simulink model "Marine_LocoMotive_UAV_est_git"  (R2018a)
settings: Solver=ode4  StartTime=0.0  StopTime=40  FixedStep=T  MaxStep=2*T  MinStep=T  RelTol=1e-4
values from neighbouring files (symbols this model uses):
  a_11 = 0.05*m_b    (= 0.625)    [Marine_LocoMotive_UAV_est_git_parameters.m]    (also in Marine_LocoMotive_UAV_medium_est_git_parameters.m = 1.6875; heave_dynamics_chart.m)
  a_33 = m_b    (= 12.5)    [Marine_LocoMotive_UAV_est_git_parameters.m]    (also in Marine_LocoMotive_UAV_medium_est_git_parameters.m = 33.75; heave_dynamics_chart.m)
  A_w = 1*3.3/2    (= 1.65)    [Marine_LocoMotive_UAV_est_git_parameters.m]    (also in Marine_LocoMotive_UAV_medium_est_git_parameters.m = 0.6)
  A_w2 = 1*1.2/2    (= 0.6)    [Marine_LocoMotive_UAV_est_git_parameters.m]    (also in Marine_LocoMotive_UAV_medium_est_git_parameters.m = 0.305)
  Ac = 0.0331    [Marine_LocoMotive_UAV_est_git_parameters.m]    (also in Marine_LocoMotive_UAV_medium_est_git_parameters.m = 0.422)
  alpha_bar = pi/4    (= 0.785398163397)    [Marine_LocoMotive_UAV_est_git_parameters.m]    (also in Marine_LocoMotive_UAV_medium_est_git_parameters.m; heave_dynamics_chart.m = pi/4*sign(V_bar(j)))
  Am = sysd.denominator{1}    [Marine_LocoMotive_UAV_est_git_parameters.m]    (also in Marine_LocoMotive_UAV_medium_est_git_parameters.m)
  Am1_LPF = sysd.denominator{1}    [Marine_LocoMotive_UAV_est_git_parameters.m]    (also in Marine_LocoMotive_UAV_medium_est_git_parameters.m)
  Am2_LPF = sysd.denominator{1}    [Marine_LocoMotive_UAV_est_git_parameters.m]    (also in Marine_LocoMotive_UAV_medium_est_git_parameters.m)
  Am_asw_LPF = sysd.denominator{1}    [Marine_LocoMotive_UAV_est_git_parameters.m]    (also in Marine_LocoMotive_UAV_medium_est_git_parameters.m)
  Am_coup_LPF = sysd.denominator{1}    [Marine_LocoMotive_UAV_est_git_parameters.m]    (also in Marine_LocoMotive_UAV_medium_est_git_parameters.m)
  Am_fast_coup_LPF = sysd.denominator{1}    [Marine_LocoMotive_UAV_est_git_parameters.m]    (also in Marine_LocoMotive_UAV_medium_est_git_parameters.m)
  Am_rdeL_LPF = sysd.denominator{1}    [Marine_LocoMotive_UAV_est_git_parameters.m]    (also in Marine_LocoMotive_UAV_medium_est_git_parameters.m)
  Am_reL_LPF = sysd.denominator{1}    [Marine_LocoMotive_UAV_est_git_parameters.m]    (also in Marine_LocoMotive_UAV_medium_est_git_parameters.m)
  Am_rref20_LPF = sysd.denominator{1}    [Marine_LocoMotive_UAV_est_git_parameters.m]    (also in Marine_LocoMotive_UAV_medium_est_git_parameters.m)
  Am_rref_LPF = sysd.denominator{1}    [Marine_LocoMotive_UAV_est_git_parameters.m]    (also in Marine_LocoMotive_UAV_medium_est_git_parameters.m)
  AmAlpha_LPF = sysd.denominator{1}    [Marine_LocoMotive_UAV_est_git_parameters.m]    (also in Marine_LocoMotive_UAV_medium_est_git_parameters.m)
  Amp_sf = 3    [Marine_LocoMotive_UAV_est_git_parameters.m]    (also in Marine_LocoMotive_UAV_medium_est_git_parameters.m)
  Amp_sf_rp = 0.05*m_u*g    (= 0.8829)    [Marine_LocoMotive_UAV_est_git_parameters.m]    (also in Marine_LocoMotive_UAV_medium_est_git_parameters.m = 9.56475)
  AmV_LPF = sysd.denominator{1}    [Marine_LocoMotive_UAV_est_git_parameters.m]    (also in Marine_LocoMotive_UAV_medium_est_git_parameters.m)
  AmZ_LPF = sysd.denominator{1}    [Marine_LocoMotive_UAV_est_git_parameters.m]    (also in Marine_LocoMotive_UAV_medium_est_git_parameters.m)
  b_11 = 0    [Marine_LocoMotive_UAV_est_git_parameters.m]    (also in Marine_LocoMotive_UAV_medium_est_git_parameters.m; heave_dynamics_chart.m)
  b_33 = 2*m_b*omega_h    (= 19.6349540849)    [Marine_LocoMotive_UAV_est_git_parameters.m]    (also in Marine_LocoMotive_UAV_medium_est_git_parameters.m = 84.8230016469; buoyancy_calc.m = 4.18879020479; heave_dynamics_chart.m = 2*m_b*omega_h)
  Bm = sysd.numerator{1}    [Marine_LocoMotive_UAV_est_git_parameters.m]    (also in Marine_LocoMotive_UAV_medium_est_git_parameters.m)
  Bm1_LPF = sysd.numerator{1}    [Marine_LocoMotive_UAV_est_git_parameters.m]    (also in Marine_LocoMotive_UAV_medium_est_git_parameters.m)
  Bm2_LPF = sysd.numerator{1}    [Marine_LocoMotive_UAV_est_git_parameters.m]    (also in Marine_LocoMotive_UAV_medium_est_git_parameters.m)
  Bm_asw_LPF = sysd.numerator{1}    [Marine_LocoMotive_UAV_est_git_parameters.m]    (also in Marine_LocoMotive_UAV_medium_est_git_parameters.m)
  Bm_coup_LPF = sysd.numerator{1}    [Marine_LocoMotive_UAV_est_git_parameters.m]    (also in Marine_LocoMotive_UAV_medium_est_git_parameters.m)
  Bm_fast_coup_LPF = sysd.numerator{1}    [Marine_LocoMotive_UAV_est_git_parameters.m]    (also in Marine_LocoMotive_UAV_medium_est_git_parameters.m)
  Bm_rdeL_LPF = sysd.numerator{1}    [Marine_LocoMotive_UAV_est_git_parameters.m]    (also in Marine_LocoMotive_UAV_medium_est_git_parameters.m)
  Bm_reL_LPF = sysd.numerator{1}    [Marine_LocoMotive_UAV_est_git_parameters.m]    (also in Marine_LocoMotive_UAV_medium_est_git_parameters.m)
  Bm_rref20_LPF = sysd.numerator{1}    [Marine_LocoMotive_UAV_est_git_parameters.m]    (also in Marine_LocoMotive_UAV_medium_est_git_parameters.m)
  Bm_rref_LPF = sysd.numerator{1}    [Marine_LocoMotive_UAV_est_git_parameters.m]    (also in Marine_LocoMotive_UAV_medium_est_git_parameters.m)
  BmAlpha_LPF = sysd.numerator{1}    [Marine_LocoMotive_UAV_est_git_parameters.m]    (also in Marine_LocoMotive_UAV_medium_est_git_parameters.m)
  BmV_LPF = sysd.numerator{1}    [Marine_LocoMotive_UAV_est_git_parameters.m]    (also in Marine_LocoMotive_UAV_medium_est_git_parameters.m)
  BmZ_LPF = sysd.numerator{1}    [Marine_LocoMotive_UAV_est_git_parameters.m]    (also in Marine_LocoMotive_UAV_medium_est_git_parameters.m)
  C_S = [5;9]*10^-3    [Marine_LocoMotive_UAV_est_git_parameters.m]    (also in Marine_LocoMotive_UAV_medium_est_git_parameters.m; heave_dynamics_chart.m = 0.075/(log10(Re)-2)^2)
  Cd_u = 0.2    [Marine_LocoMotive_UAV_est_git_parameters.m]    (also in Marine_LocoMotive_UAV_medium_est_git_parameters.m)
  D_x = b_11 + D_s(1)    [Marine_LocoMotive_UAV_est_git_parameters.m]    (also in Marine_LocoMotive_UAV_medium_est_git_parameters.m; heave_dynamics_chart.m = b_11 + D_s(i,j))
  D_z = b_33 + D_s(2)    [Marine_LocoMotive_UAV_est_git_parameters.m]    (also in Marine_LocoMotive_UAV_medium_est_git_parameters.m; heave_dynamics_chart.m)
  dc_M_p = 6.7    [Marine_LocoMotive_UAV_est_git_parameters.m]    (also in Marine_LocoMotive_UAV_medium_est_git_parameters.m)
  Delta_h = (A_im/A_b-0.5)*h_b    (= -0.0625)    [Marine_LocoMotive_UAV_est_git_parameters.m]    (also in Marine_LocoMotive_UAV_medium_est_git_parameters.m = -0.075; heave_dynamics_chart.m)
  eps_V = 0.1    [Marine_LocoMotive_UAV_est_git_parameters.m]    (also in Marine_LocoMotive_UAV_medium_est_git_parameters.m)
  epsilon_1 = 5    [Marine_LocoMotive_UAV_est_git_parameters.m]    (also in Marine_LocoMotive_UAV_medium_est_git_parameters.m)
  epsilon_e_u1 = 0.05    [Marine_LocoMotive_UAV_est_git_parameters.m]    (also in Marine_LocoMotive_UAV_medium_est_git_parameters.m)
  epsilon_w = 0    [Marine_LocoMotive_UAV_est_git_parameters.m]    (also in Marine_LocoMotive_UAV_medium_est_git_parameters.m)
  epsilon_w2 = pi    (= 3.14159265359)    [Marine_LocoMotive_UAV_est_git_parameters.m]    (also in Marine_LocoMotive_UAV_medium_est_git_parameters.m)
  g = 9.81    [Marine_LocoMotive_UAV_est_git_parameters.m]    (also in Marine_LocoMotive_UAV_medium_est_git_parameters.m; heave_dynamics_chart.m)
  gamma_d_p = (2*0.3/0.03*2*0.2*12/4)/10    (= 2.4)    [Marine_LocoMotive_UAV_est_git_parameters.m]    (also in Marine_LocoMotive_UAV_medium_est_git_parameters.m)
  H = 10    [Marine_LocoMotive_UAV_est_git_parameters.m]    (also in Marine_LocoMotive_UAV_medium_est_git_parameters.m)
  h_b = 0.25    [Marine_LocoMotive_UAV_est_git_parameters.m]    (also in Marine_LocoMotive_UAV_medium_est_git_parameters.m = 0.3; buoyancy_calc.m = 0.15; heave_dynamics_chart.m)
  J_b = m_b*h_b*l_b/12    (= 0.208333333333)    [Marine_LocoMotive_UAV_est_git_parameters.m]    (also in Marine_LocoMotive_UAV_medium_est_git_parameters.m = 1.265625; heave_dynamics_chart.m)
  J_u = 0.03    [Marine_LocoMotive_UAV_est_git_parameters.m]    (also in Marine_LocoMotive_UAV_medium_est_git_parameters.m = 1.51708333333)
  K = 40    [Marine_LocoMotive_UAV_est_git_parameters.m]    (also in Marine_LocoMotive_UAV_medium_est_git_parameters.m = 83.3333333333)
  k3 = 24    [Marine_LocoMotive_UAV_est_git_parameters.m]    (also in Marine_LocoMotive_UAV_medium_est_git_parameters.m)
  k4 = 0.8    [Marine_LocoMotive_UAV_est_git_parameters.m]    (also in Marine_LocoMotive_UAV_medium_est_git_parameters.m)
  k_w = omega_w^2/g    (= 0.0628797426165)    [Marine_LocoMotive_UAV_est_git_parameters.m]    (also in Marine_LocoMotive_UAV_medium_est_git_parameters.m = 0.160972141098; heave_dynamics_chart.m = omega_w^2/g)
  k_w2 = omega_w2^2/g    (= 0.160972141098)    [Marine_LocoMotive_UAV_est_git_parameters.m]    (also in Marine_LocoMotive_UAV_medium_est_git_parameters.m = 0.251518970466)
  kd_a = 5.6    [Marine_LocoMotive_UAV_est_git_parameters.m]    (also in Marine_LocoMotive_UAV_medium_est_git_parameters.m)
  kd_r = 19.5    [Marine_LocoMotive_UAV_est_git_parameters.m]    (also in Marine_LocoMotive_UAV_medium_est_git_parameters.m)
  kd_t = 10    [Marine_LocoMotive_UAV_est_git_parameters.m]    (also in Marine_LocoMotive_UAV_medium_est_git_parameters.m = 25)
  kd_x = 5    [Marine_LocoMotive_UAV_est_git_parameters.m]    (also in Marine_LocoMotive_UAV_medium_est_git_parameters.m)
  kd_z = 2    [Marine_LocoMotive_UAV_est_git_parameters.m]    (also in Marine_LocoMotive_UAV_medium_est_git_parameters.m)
  ki_a = 1.6    [Marine_LocoMotive_UAV_est_git_parameters.m]    (also in Marine_LocoMotive_UAV_medium_est_git_parameters.m)
  ki_r = 9    [Marine_LocoMotive_UAV_est_git_parameters.m]    (also in Marine_LocoMotive_UAV_medium_est_git_parameters.m)
  ki_T = 12    [Marine_LocoMotive_UAV_est_git_parameters.m]    (also in Marine_LocoMotive_UAV_medium_est_git_parameters.m)
  ki_x = 1.2    [Marine_LocoMotive_UAV_est_git_parameters.m]    (also in Marine_LocoMotive_UAV_medium_est_git_parameters.m)
  ki_z = 1    [Marine_LocoMotive_UAV_est_git_parameters.m]    (also in Marine_LocoMotive_UAV_medium_est_git_parameters.m)
  kp_a = 9.6    [Marine_LocoMotive_UAV_est_git_parameters.m]    (also in Marine_LocoMotive_UAV_medium_est_git_parameters.m)
  kp_r = 45    [Marine_LocoMotive_UAV_est_git_parameters.m]    (also in Marine_LocoMotive_UAV_medium_est_git_parameters.m)
  kp_t = 20    [Marine_LocoMotive_UAV_est_git_parameters.m]    (also in Marine_LocoMotive_UAV_medium_est_git_parameters.m = 50)
  kp_T = 25    [Marine_LocoMotive_UAV_est_git_parameters.m]    (also in Marine_LocoMotive_UAV_medium_est_git_parameters.m)
  kp_x = 7    [Marine_LocoMotive_UAV_est_git_parameters.m]    (also in Marine_LocoMotive_UAV_medium_est_git_parameters.m)
  kp_z = 3    [Marine_LocoMotive_UAV_est_git_parameters.m]    (also in Marine_LocoMotive_UAV_medium_est_git_parameters.m)
  L = 0.2    [Marine_LocoMotive_UAV_est_git_parameters.m]    (also in Marine_LocoMotive_UAV_medium_est_git_parameters.m = 0.8)
  l_b = 0.8    [Marine_LocoMotive_UAV_est_git_parameters.m]    (also in Marine_LocoMotive_UAV_medium_est_git_parameters.m = 1.5; buoyancy_calc.m = 0.5; heave_dynamics_chart.m)
  Lc_0 = 7    [Marine_LocoMotive_UAV_est_git_parameters.m]    (also in Marine_LocoMotive_UAV_medium_est_git_parameters.m = 20)
  LIMIT_CMD_PITCH = 45*pi/180    (= 0.785398163397)    [Marine_LocoMotive_UAV_est_git_parameters.m]    (also in Marine_LocoMotive_UAV_medium_est_git_parameters.m)
  LIMIT_uCMD_HEIGHT = 0.9*n_motors*K    (= 144)    [Marine_LocoMotive_UAV_est_git_parameters.m]    (also in Marine_LocoMotive_UAV_medium_est_git_parameters.m = 450)
  m_b = rho_w*Vol_b/4    (= 12.5)    [Marine_LocoMotive_UAV_est_git_parameters.m]    (also in Marine_LocoMotive_UAV_medium_est_git_parameters.m = 33.75; buoyancy_calc.m = 5; heave_dynamics_chart.m)
  m_u = 1.8    [Marine_LocoMotive_UAV_est_git_parameters.m]    (also in Marine_LocoMotive_UAV_medium_est_git_parameters.m = 19.5)
  min_sf = 5    [Marine_LocoMotive_UAV_est_git_parameters.m]    (also in Marine_LocoMotive_UAV_medium_est_git_parameters.m)
  min_sf_rp = 0.35*m_u*g    (= 6.1803)    [Marine_LocoMotive_UAV_est_git_parameters.m]    (also in Marine_LocoMotive_UAV_medium_est_git_parameters.m = 66.95325)
  n_motors = 4    [Marine_LocoMotive_UAV_est_git_parameters.m]    (also in Marine_LocoMotive_UAV_medium_est_git_parameters.m = 6)
  nu_w = 1.787*10^-6    (= 1.787e-06)    [Marine_LocoMotive_UAV_est_git_parameters.m]    (also in Marine_LocoMotive_UAV_medium_est_git_parameters.m; buoyancy_calc.m; heave_dynamics_chart.m)
  omega_w = 2*pi/T_w    (= 0.785398163397)    [Marine_LocoMotive_UAV_est_git_parameters.m]    (also in Marine_LocoMotive_UAV_medium_est_git_parameters.m = 1.25663706144; heave_dynamics_chart.m = 2*pi/T_i)
  omega_w2 = 2*pi/T_w2    (= 1.25663706144)    [Marine_LocoMotive_UAV_est_git_parameters.m]    (also in Marine_LocoMotive_UAV_medium_est_git_parameters.m = 1.57079632679)
  r_0 = sqrt( (X0_b(1) - X0_u(1))^2 +(X0_b(2) - X0_u(2))^2 )    [Marine_LocoMotive_UAV_est_git_parameters.m]    (also in Marine_LocoMotive_UAV_medium_est_git_parameters.m)
  R_b = 0.1    [buoyancy_calc.m]
  r_bar = Lc_0-0.3    (= 6.7)    [Marine_LocoMotive_UAV_est_git_parameters.m]    (also in Marine_LocoMotive_UAV_medium_est_git_parameters.m = 19.7)
  r_min = (zu_bar-H)-0.2    [Marine_LocoMotive_UAV_est_git_parameters.m]    (also in Marine_LocoMotive_UAV_medium_est_git_parameters.m)
  rho_a = 1.225    [Marine_LocoMotive_UAV_est_git_parameters.m]    (also in Marine_LocoMotive_UAV_medium_est_git_parameters.m)
  rho_w = 1000    [Marine_LocoMotive_UAV_est_git_parameters.m]    (also in Marine_LocoMotive_UAV_medium_est_git_parameters.m; buoyancy_calc.m; heave_dynamics_chart.m)
  T = 1/500    (= 0.002)    [Marine_LocoMotive_UAV_est_git_parameters.m]    (also in Marine_LocoMotive_UAV_medium_est_git_parameters.m)
  T_init = 10    [Marine_LocoMotive_UAV_est_git_parameters.m]    (also in Marine_LocoMotive_UAV_medium_est_git_parameters.m)
  Theta0 = 0    [Marine_LocoMotive_UAV_est_git_parameters.m]    (also in Marine_LocoMotive_UAV_medium_est_git_parameters.m)
  torque_corr = 2*cosd(60)+1    [Marine_LocoMotive_UAV_est_git_parameters.m]    (also in Marine_LocoMotive_UAV_medium_est_git_parameters.m)
  u_s = w_dir*A_w^2*omega_w*k_w*exp(2*k_w*(-Delta_h/2))    [Marine_LocoMotive_UAV_est_git_parameters.m]    (also in Marine_LocoMotive_UAV_medium_est_git_parameters.m)
  u_s2 = w_dir2*A_w2^2*omega_w2*k_w2*exp(2*k_w2*(-Delta_h/2))    [Marine_LocoMotive_UAV_est_git_parameters.m]    (also in Marine_LocoMotive_UAV_medium_est_git_parameters.m)
  u_t = -1*0.5*1    (= -0.5)    [Marine_LocoMotive_UAV_est_git_parameters.m]    (also in Marine_LocoMotive_UAV_medium_est_git_parameters.m)
  u_w = 0*0.2    (= 0)    [Marine_LocoMotive_UAV_est_git_parameters.m]    (also in Marine_LocoMotive_UAV_medium_est_git_parameters.m)
  V0_b = [u_t+u_w+u_s+v_x_w, v_z_w].*[1 1]    [Marine_LocoMotive_UAV_est_git_parameters.m]    (also in Marine_LocoMotive_UAV_medium_est_git_parameters.m = [u_t+u_w+u_s+v_x_w, v_z_w])
  V0_u = V0_b    [Marine_LocoMotive_UAV_est_git_parameters.m]    (also in Marine_LocoMotive_UAV_medium_est_git_parameters.m = [0 0])
  V_bar = 4    [Marine_LocoMotive_UAV_est_git_parameters.m]    (also in Marine_LocoMotive_UAV_medium_est_git_parameters.m; heave_dynamics_chart.m = [-20:0.1:20]')
  Vol_b = A_b*l_b    (= 0.05)    [Marine_LocoMotive_UAV_est_git_parameters.m]    (also in Marine_LocoMotive_UAV_medium_est_git_parameters.m = 0.135; heave_dynamics_chart.m)
  w_dir = 1    [Marine_LocoMotive_UAV_est_git_parameters.m]    (also in Marine_LocoMotive_UAV_medium_est_git_parameters.m; heave_dynamics_chart.m)
  w_dir2 = 1    [Marine_LocoMotive_UAV_est_git_parameters.m]    (also in Marine_LocoMotive_UAV_medium_est_git_parameters.m)
  X0_b = [0,H-Delta_h]    [Marine_LocoMotive_UAV_est_git_parameters.m]    (also in Marine_LocoMotive_UAV_medium_est_git_parameters.m)
  X0_u = X0_b + [3/7 3/7]*Lc_0    [Marine_LocoMotive_UAV_est_git_parameters.m]    (also in Marine_LocoMotive_UAV_medium_est_git_parameters.m)
  zu_bar = X0_b(2) + Lc_0*sin(alpha_bar_0)    [Marine_LocoMotive_UAV_est_git_parameters.m]    (also in Marine_LocoMotive_UAV_medium_est_git_parameters.m)
undefined symbols (not defined in the file or in its folder): Am_HPF, Am_LPF, Am_LPF2, an1, an1_v, an2, an3, Bm_HPF, Bm_LPF, Bm_LPF2, bn1, bn1_v, bn2, bn3, DiscIntNeverNeededParam, F, Light, magnitude, MIL, OMEGA_FILTER_OUTER, Tc, Tg, Tn, Ts, Tsc, Tz, X_GPS_offset
libraries: simulink x55, simulink_extras x9, aerolibwind2 x2
(part 7 of 9)

== system Marine_LocoMotive_UAV_est_git/Quadrotor+buoy/3-DOF equations of motion Earth frame/Quadrotor Dynamics Outer-Loop/Integrator while decoupled ==
  acc : Inport
  X dot init : Inport  Port=2
  X init : Inport  Port=3
  X123 : Inport  Port=4
  reset : Inport  Port=5
  Enable : EnablePort
  Bias : Bias  Bias=Lc_0
  Bias1 : Bias  Bias=Lc_0
  Bias2 : Bias  Bias=-Lc_0
  Bias3 : Bias  Bias=-Lc_0
  Saturation Dynamic : simulink/Discontinuities/Saturation Dynamic  OutMin=[]  OutMax=[]  OutDataTypeStr=Inherit: Same as second input  OutDataType=fixdt(1, 16)  OutScaling=2^-10  DoSatur=off
  Selector : Selector  InputPortWidth=3  IndexOptions=Index vector (dialog)  Indices=1  OutputSizes=1
  Selector1 : Selector  InputPortWidth=3  IndexOptions=Index vector (dialog)  Indices=2  OutputSizes=1
  Vector Concatenate : Concatenate
  Vector Concatenate1 : Concatenate
  Vector Concatenate2 : Concatenate
  Xu : DiscreteIntegrator  IntegratorMethod=Integration: Backward Euler  ExternalReset=level  InitialConditionSource=external  InitialCondition=theta_q_ini  SampleTime=-1  LimitOutput=on  StateName=theta  ICPrevOutput=DiscIntNeverNeededParam  ICPrevScaledInput=DiscIntNeverNeededParam
  dot(Xu) : DiscreteIntegrator  IntegratorMethod=Integration: Backward Euler  gainval=1  ExternalReset=level  InitialConditionSource=external  SampleTime=-1  ICPrevOutput=DiscIntNeverNeededParam  ICPrevScaledInput=DiscIntNeverNeededParam
  theta u{1..11} (11 alike) : Scope
  "dot(Xu) " : Outport
  "Xu " : Outport  Port=2
  wires:
  X dot init/1 -> theta u5/1, dot(Xu)/3
  Xu/1 -> theta u6/1, Vector Concatenate2/1, Saturation Dynamic/2
  X init/1 -> theta u7/1, Xu/3
  Saturation Dynamic/1 -> Vector Concatenate2/2, "Xu "/1
  X123/1 -> Selector1/1, Selector/1
  Selector/1 -> Bias2/1, Bias/1
  Bias/1 -> Vector Concatenate/1
  Bias1/1 -> theta u11/1, Vector Concatenate/2
  Bias2/1 -> Vector Concatenate1/1
  Bias3/1 -> Vector Concatenate1/2
  Vector Concatenate1/1 -> theta u10/1, Saturation Dynamic/3
  Vector Concatenate2/1 -> theta u3/1
  Vector Concatenate/1 -> theta u9/1, Saturation Dynamic/1
  dot(Xu)/1 -> Xu/1, theta u1/1, "dot(Xu) "/1
  reset/1 -> theta u2/1, dot(Xu)/2, Xu/2
  acc/1 -> theta u4/1, dot(Xu)/1
  Selector1/1 -> theta u8/1, Bias3/1, Bias1/1

== system Marine_LocoMotive_UAV_est_git/Quadrotor+buoy/3-DOF equations of motion Earth frame/Quadrotor Dynamics Outer-Loop/Subsystem ==
  u1 : Inport
  theta_u : Inport  Port=2
  Product1 : Product  Inputs=**  SaturateOnIntegerOverflow=on  InputSameDT=on  OutDataTypeStr=Inherit: Same as first input
  Product7 : Product  Inputs=**  SaturateOnIntegerOverflow=on  InputSameDT=on  OutDataTypeStr=Inherit: Same as first input
  Trigonometric Function1 : Trigonometry  Operator=sincos
  Vector Concatenate3 : Concatenate
  tau_u : Outport
  wires:
  Product7/1 -> Vector Concatenate3/2
  Product1/1 -> Vector Concatenate3/1
  u1/1 -> Product7/2, Product1/1
  theta_u/1 -> Trigonometric Function1/1
  Trigonometric Function1/1 -> Product1/2
  Trigonometric Function1/2 -> Product7/1
  Vector Concatenate3/1 -> tau_u/1

== system Marine_LocoMotive_UAV_est_git/Quadrotor+buoy/3-DOF equations of motion Earth frame/Quadrotor Dynamics Outer-Loop/get initial UAV states for the decoupled dynamics ==
  X : Inport
  Xdot : Inport  Port=2
  Trigger : TriggerPort  TriggerType=falling  VariantControl=Variant
  Xu_init : Outport
  Vu_init : Outport  Port=2
  wires:
  X/1 -> Xu_init/1
  Xdot/1 -> Vu_init/1

== system Marine_LocoMotive_UAV_est_git/Quadrotor+buoy/3-DOF equations of motion Earth frame/Quadrotor Dynamics Outer-Loop/quadrotor position from relative buoy-UAV position ==
  X123 : Inport
  Xdot123 : Inport  Port=2
  Xddot123 : Inport  Port=3
  Enable : EnablePort
  Demux : Demux  Outputs=3
  Demux1 : Demux  Outputs=3
  Demux2 : Demux  Outputs=3
  Gain{,1..3} (4 alike) : Gain  Gain=L
  Product : Product
  Product1 : Product
  Product2 : Product
  Product3 : Product  Multiplication=Matrix(*)
  Sum : Sum  Inputs=|++
  Sum1 : Sum  Inputs=|++
  Sum2 : Sum  Inputs=-+|
  Sum3 : Sum  Inputs=++|
  Sum4 : Sum  Inputs=++|
  Trigonometric Function : Trigonometry  Operator=sincos
  Vector Concatenate{1..4} (4 alike) : Concatenate
  "rotation matrix R " : Subsystem
  theta u{1..6} (6 alike) : Scope
  Xu : Outport
  Xu_dot : Outport  Port=2
  Xu_ddot1 : Outport  Port=3
  wires:
  Trigonometric Function/2 -> Gain3/1
  Trigonometric Function/1 -> Gain/1
  Demux/3 -> "rotation matrix R "/1(angle (rad)), theta u2/1, Trigonometric Function/1  "alpha"
  Sum1/1 -> Vector Concatenate3/2
  Vector Concatenate3/1 -> theta u4/1, Xu/1
  Gain3/1 -> Product1/1, Sum/2
  Demux/2 -> theta u3/1, Sum1/1  "z_b"
  Gain/1 -> Product/1, Sum1/2
  Sum/1 -> Vector Concatenate3/1
  X123/1 -> Demux/1
  Demux/1 -> theta u1/1, Sum/1  "x_b"
  "rotation matrix R "/1(R) -> Product3/1
  Xdot123/1 -> Demux1/1
  Sum2/1 -> Vector Concatenate1/1
  Vector Concatenate1/1 -> theta u5/1, Xu_dot/1
  Sum3/1 -> Vector Concatenate1/2
  Demux1/1 -> Sum2/2
  Demux1/2 -> Sum3/2
  Product/1 -> Sum2/1
  Product1/1 -> Sum3/1
  Xddot123/1 -> Demux2/1
  Product2/1 -> Gain1/1
  Demux1/3 -> Product2/2, Product2/1, Product1/2, Product/2
  Demux2/3 -> Gain2/1
  Gain2/1 -> Vector Concatenate2/2
  Gain1/1 -> Vector Concatenate2/1
  Vector Concatenate2/1 -> Product3/2
  Sum4/1 -> theta u6/1, Xu_ddot1/1
  Demux2/1 -> Vector Concatenate4/1
  Demux2/2 -> Vector Concatenate4/2
  Vector Concatenate4/1 -> Sum4/2
  Product3/1 -> Sum4/1

== system Marine_LocoMotive_UAV_est_git/Quadrotor+buoy/3-DOF equations of motion Earth frame/Quadrotor Dynamics Outer-Loop/rotation matrix R transpose ==
  angle (rad) : Inport
  Gain : Gain  Gain=-1
  Signal Specification1 : SignalSpecification  Dimensions=2
  Signal Specification2 : SignalSpecification  Dimensions=2
  Trigonometric Function1 : Trigonometry  Operator=sincos
  Vector Concatenate1 : Concatenate  Mode=Multidimensional array  ConcatenateDimension=2
  Vector Concatenate2 : Concatenate
  Vector Concatenate3 : Concatenate
  R : Outport
  wires:
  Signal Specification2/1 -> Vector Concatenate1/2
  Signal Specification1/1 -> Vector Concatenate1/1
  Vector Concatenate1/1 -> R/1
  Vector Concatenate2/1 -> Signal Specification1/1
  Vector Concatenate3/1 -> Signal Specification2/1
  angle (rad)/1 -> Trigonometric Function1/1
  Trigonometric Function1/2 -> Vector Concatenate3/2, Vector Concatenate2/1
  Trigonometric Function1/1 -> Vector Concatenate3/1, Gain/1
  Gain/1 -> Vector Concatenate2/2

== system Marine_LocoMotive_UAV_est_git/Quadrotor+buoy/3-DOF equations of motion Earth frame/Tension from UAV, X and r directions/Tension from UAV, X and r directions ==
  alpha : Inport
  theta_u : Inport  Port=2
  u1 : Inport  Port=3
  Xu_ddot : Inport  Port=4
  Add3 : Sum  Inputs=+--
  Constant : Constant  Value=m_u*g
  Gain14 : Gain
  Gain15 : Gain  Gain=m_u
  Product12 : Product
  Product9 : Product  Inputs=*/
  Trigonometric Function6 : Trigonometry
  Trigonometric Function8 : Trigonometry  Operator=cos
  x_ddot1 : Selector  InputPortWidth=2  IndexOptions=Index vector (dialog)  Indices=2  OutputSizes=1
  "T, from x simple" : Outport
  wires:
  Product9/1 -> "T, from x simple"/1
  Add3/1 -> Product9/1
  Gain14/1 -> Add3/1
  Trigonometric Function8/1 -> Product12/1
  u1/1 -> Product12/2
  alpha/1 -> Trigonometric Function6/1
  Product12/1 -> Gain14/1
  x_ddot1/1 -> Gain15/1
  Trigonometric Function6/1 -> Product9/2
  Xu_ddot/1 -> x_ddot1/1
  theta_u/1 -> Trigonometric Function8/1
  Gain15/1 -> Add3/2
  Constant/1 -> Add3/3

== system Marine_LocoMotive_UAV_est_git/Quadrotor+buoy/3-DOF equations of motion Earth frame/azimuthal dynamics/Coupled System's azimuthal dynamics ==
  alpha dc : Inport
  alpha_dot dc : Inport  Port=2
  coupled : Inport  Port=3
  alpha_ddot : Inport  Port=4
  recouple : Inport  Port=5
    alpha{,1..5} (6 alike) : Scope
  Clock : Clock
  Constant : Constant  Value=0
  Delay : Delay  DelayLength=1
  IC1 : InitialCondition  Value=alpha_0
  IC2 : InitialCondition  Value=0
  IC3 : InitialCondition  Value=alpha_0
  Logical Operator1 : Logic  Operator=NOT  AllPortsSameDT=off  OutDataTypeStr=boolean
  Switch : Switch  Criteria=u2 > Threshold  Threshold=2*T
  "T, r,xu,xb1" : Scope
  "T, r,xu,xb9" : Scope
  azimuth angle dynamics in the coupled system : Subsystem  TreatAsAtomicUnit=on
  get initial azimuth angle for the coupled dynamics : Subsystem  TreatAsAtomicUnit=on
  alpha coupled : Outport
  alpha dot coupled : Outport  Port=2
  wires:
  alpha_ddot/1 -> azimuth angle dynamics in the coupled system/1(alpha_ddot)
  coupled/1 -> azimuth angle dynamics in the coupled system/Enable, Logical Operator1/1
  azimuth angle dynamics in the coupled system/1("alpha ") -> IC3/1
  azimuth angle dynamics in the coupled system/2(alpha dot) -> alpha dot coupled/1
  alpha dc/1 -> "  alpha2"/1, get initial azimuth angle for the coupled dynamics/1(alpha decoupled)
  alpha_dot dc/1 -> "  alpha1"/1, get initial azimuth angle for the coupled dynamics/2(alpha dot decoupled)
  get initial azimuth angle for the coupled dynamics/1(alpha init) -> "  alpha3"/1, IC1/1
  IC1/1 -> "  alpha4"/1, azimuth angle dynamics in the coupled system/2(alpha init)
  IC2/1 -> "  alpha5"/1, azimuth angle dynamics in the coupled system/3(alpha dot init)
  get initial azimuth angle for the coupled dynamics/2(alpha dot init) -> IC2/1
  recouple/1 -> "  alpha"/1, get initial azimuth angle for the coupled dynamics/Trigger
  Logical Operator1/1 -> Delay/1
  Delay/1 -> Switch/1, "T, r,xu,xb1"/1
  Clock/1 -> Switch/2
  Switch/1 -> "T, r,xu,xb9"/1, azimuth angle dynamics in the coupled system/4(reset)
  Constant/1 -> Switch/3
  IC3/1 -> alpha coupled/1

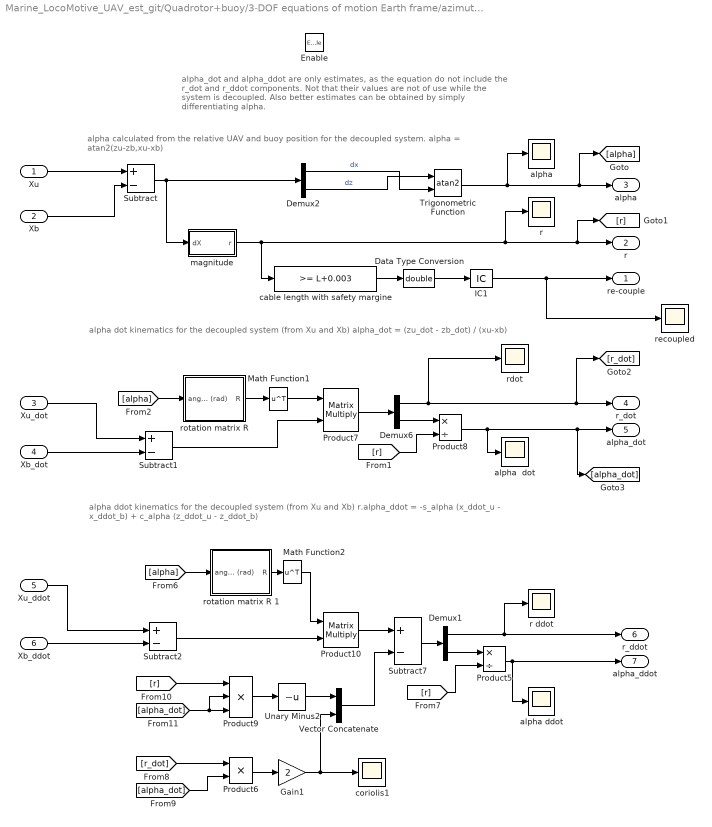
== system Marine_LocoMotive_UAV_est_git/Quadrotor+buoy/3-DOF equations of motion Earth frame/azimuthal dynamics/Decoupled System's azimuthal dynamics ==
  note: alpha_dot and alpha_ddot are only estimates,
      | as the equation do not include the r_dot and r_ddot components.
      | Not that their values are not of use while the system is decoupled.
      | Also better estimates can be obtained by simply differentiating alpha.
  note: alpha dot kinematics for the decoupled system (from Xu and Xb)
      | alpha_dot =  (zu_dot - zb_dot) / (xu-xb)
  note: alpha calculated from the relative UAV and buoy position for the decoupled system.
      | alpha = atan2(zu-zb,xu-xb)
  note: alpha ddot kinematics for the decoupled system (from Xu and Xb)
      | r.alpha_ddot = -s_alpha (x_ddot_u - x_ddot_b) + c_alpha (z_ddot_u - z_ddot_b)
  Xu : Inport
  Xb : Inport  Port=2
  Xu_dot : Inport  Port=3
  Xb_dot : Inport  Port=4
  Xu_ddot : Inport  Port=5
  Xb_ddot : Inport  Port=6
  Enable : EnablePort
  " r" : Scope
  Data Type Conversion : DataTypeConversion  OutDataTypeStr=double
  Demux1 : Demux  Outputs=2
  Demux2 : Demux  Outputs=2
  Demux6 : Demux  Outputs=2
  Gain1 : Gain  Gain=2
  IC1 : InitialCondition  Value=0
  Math Function1 : Math  Operator=transpose  SaturateOnIntegerOverflow=on
  Math Function2 : Math  Operator=transpose  SaturateOnIntegerOverflow=on
  Product10 : Product  Multiplication=Matrix(*)
  Product5 : Product  Inputs=*/
  Product6 : Product
  Product7 : Product  Multiplication=Matrix(*)
  Product8 : Product  Inputs=*/
  Product9 : Product  Inputs=3
  Subtract{,1..2,7} (4 alike) : Sum  Inputs=+-
  Trigonometric Function : Trigonometry  Operator=atan2
  Unary Minus2 : UnaryMinus
  Vector Concatenate : Concatenate
  "alpha     " : Scope
  alpha  dot : Scope
  alpha ddot : Scope
  cable length with safety margine : simulink/Logic and Bit Operations/Compare To Constant  relop=>=  const=L+0.003  OutDataTypeStr=boolean
  coriolis1 : Scope
  magnitude : Subsystem
  r ddot : Scope
  rdot : Scope
  recoupled : Scope
  "rotation matrix R " : Subsystem
  rotation matrix R 1 : Subsystem
  re-couple : Outport  OutputWhenDisabled=reset  InitialOutput=0
  r : Outport  Port=2
  alpha : Outport  Port=3
  r_dot : Outport  Port=4
  alpha_dot : Outport  Port=5
  r_ddot : Outport  Port=6
  alpha_ddot : Outport  Port=7
  wires:
  Xu_dot/1 -> Subtract1/1
  Xb_dot/1 -> Subtract1/2
  Xu/1 -> Subtract/1
  Xb/1 -> Subtract/2
  Demux2/2 -> Trigonometric Function/1  "dz"
  Demux2/1 -> Trigonometric Function/2  "dx"
  Trigonometric Function/1 -> [alpha], alpha/1, "alpha     "/1
  Xu_ddot/1 -> Subtract2/1
  magnitude/1(r) -> cable length with safety margine/1, r/1, [r], " r"/1
  Subtract/1 -> magnitude/1(dX), Demux2/1
  cable length with safety margine/1 -> Data Type Conversion/1
  Data Type Conversion/1 -> IC1/1
  IC1/1 -> recoupled/1, re-couple/1
  [alpha] -> "rotation matrix R "/1(angle (rad))
  "rotation matrix R "/1(R) -> Math Function1/1
  Subtract1/1 -> Product7/2
  Math Function1/1 -> Product7/1
  Product7/1 -> Demux6/1
  Demux6/2 -> Product8/1
  [r] -> Product8/2
  Product8/1 -> alpha  dot/1, [alpha_dot], alpha_dot/1
  Demux6/1 -> rdot/1, [r_dot], r_dot/1
  Gain1/1 -> Vector Concatenate/2, coriolis1/1
  [r_dot] -> Product6/1
  [alpha_dot] -> Product6/2
  Product6/1 -> Gain1/1
  [r] -> Product5/2
  Xb_ddot/1 -> Subtract2/2
  rotation matrix R 1/1(R) -> Math Function2/1
  Subtract2/1 -> Product10/2
  [alpha] -> rotation matrix R 1/1(angle (rad))
  Math Function2/1 -> Product10/1
  [r] -> Product9/1
  [alpha_dot] -> Product9/2, Product9/3
  Product9/1 -> Unary Minus2/1
  Product10/1 -> Subtract7/1
  Unary Minus2/1 -> Vector Concatenate/1
  Vector Concatenate/1 -> Subtract7/2
  Subtract7/1 -> Demux1/1
  Demux1/1 -> r ddot/1, r_ddot/1
  Demux1/2 -> Product5/1
  Product5/1 -> alpha ddot/1, alpha_ddot/1

== system Marine_LocoMotive_UAV_est_git/Quadrotor+buoy/3-DOF equations of motion Earth frame/buoyancy/V_im cuboid ==
  zeta : Inport
  zb : Inport  Port=2
  Constant : Constant  Value=l_b*h_b
  Product3 : Product  SaturateOnIntegerOverflow=on  InputSameDT=on  OutDataTypeStr=Inherit: Same as first input
  Saturation : Saturate  UpperLimit=h_b/2  LowerLimit=-h_b/2
  Scope4 : Scope
  Sum : Sum  Inputs=|++
  Sum2 : Sum  Inputs=|+-  SaturateOnIntegerOverflow=on
  Vol_b/2 : Constant  Value=l_b*h_b*h_b/2
  Vol_im : Outport
  wires:
  Saturation/1 -> Product3/1
  Sum2/1 -> Saturation/1, Scope4/1  "d"
  Product3/1 -> Sum/1
  Constant/1 -> Product3/2
  Sum/1 -> Vol_im/1
  Vol_b/2/1 -> Sum/2
  zeta/1 -> Sum2/1
  zb/1 -> Sum2/2

== system Marine_LocoMotive_UAV_est_git/Quadrotor+buoy/3-DOF equations of motion Earth frame/buoyancy/f(z_b,zeta) cylinder ==
  note: This model is valid for d<=R
  zeta : Inport
  zb : Inport  Port=2
  Bias : Bias  Bias=1
  Constant : Constant  Value=R_b
  Product3 : Product  Inputs=*/  SaturateOnIntegerOverflow=on  InputSameDT=on  OutDataTypeStr=Inherit: Same as first input
  Product4 : Product  SaturateOnIntegerOverflow=on  InputSameDT=on  OutDataTypeStr=Inherit: Same as first input
  Product5 : Product  SaturateOnIntegerOverflow=on  InputSameDT=on  OutDataTypeStr=Inherit: Same as first input
  Product6 : Product  SaturateOnIntegerOverflow=on  InputSameDT=on  OutDataTypeStr=Inherit: Same as first input
  Saturation : Saturate  UpperLimit=R_b  LowerLimit=0
  Scope{1..4} (4 alike) : Scope
  Sqrt : Sqrt  SaturateOnIntegerOverflow=on
  Sum2 : Sum  Inputs=-+|  SaturateOnIntegerOverflow=on
  Sum3 : Sum  Inputs=-+|  SaturateOnIntegerOverflow=on
  Unary Minus : UnaryMinus
  acos : Trigonometry  Operator=acos
  Out1 : Outport
  wires:
  Constant/1 -> Product5/2, Product3/2
  Bias/1 -> Sqrt/1
  Product5/1 -> Scope1/1, Sum3/2
  Product4/1 -> Sum3/1
  Product6/1 -> Unary Minus/1
  Unary Minus/1 -> Bias/1
  Sum2/1 -> Scope4/1, Saturation/1  "d"
  Product3/1 -> acos/1, Product6/2, Product6/1
  Sqrt/1 -> Product4/1, Scope3/1
  acos/1 -> Product5/1
  zb/1 -> Sum2/2
  zeta/1 -> Sum2/1
  Sum3/1 -> Out1/1
  Saturation/1 -> Scope2/1, Product4/2, Product3/1

== system Marine_LocoMotive_UAV_est_git/Sensors and Filters/Data processing/Estimate Attitude/Calculate Roll and Pitch (From Acceleration Data) ==
  accel (m/s^2) [3] : Inport
  Gain1 : Gain  Commented=on  Gain=180/pi
  Gain3 : Gain
  Terminator : Terminator
  calc_roll_pitch : MATLAB Function  TreatAsAtomicUnit=on
  pitch_acc : Scope  Commented=on
  pitch_acc (rad) : Outport
  wires:
  accel (m/s^2) [3]/1 -> calc_roll_pitch/1(acc_body)
  calc_roll_pitch/2(pitch_acc) -> Gain3/1, Gain1/1
  Gain1/1 -> pitch_acc/1
  Gain3/1 -> pitch_acc (rad)/1
  calc_roll_pitch/1(roll_acc) -> Terminator/1

== system Marine_LocoMotive_UAV_est_git/Sensors and Filters/Data processing/Estimate Attitude/Notch Filter1 ==
  u : Inport
  LPF : DiscreteTransferFcn  Numerator=Bm_LPF  Denominator=Am_LPF
  Mux : Mux  Commented=on
  Mux1 : Mux  Commented=on  Inputs=2
  Notch filter 1 : DiscreteTransferFcn  Numerator=an1  Denominator=bn1  SampleTime=Tn
  Notch filter 2 : DiscreteTransferFcn  Numerator=an2  Denominator=bn2  SampleTime=Tn
  Notch filter 3 : DiscreteTransferFcn  Numerator=an3  Denominator=bn3  SampleTime=Tn
  Scope : Scope  Commented=on
  Scope1 : Scope  Commented=on
  To File : ToFile  Commented=on  Filename=P_gyro_Noisy.mat  MatrixName=P_gyro_Noisy  SaveFormat=Timeseries
  y : Outport
  q : Outport  Port=2
  wires:
  u/1 -> Mux1/1, To File/1, LPF/1
  Notch filter 2/1 -> Mux/3, Notch filter 3/1
  LPF/1 -> Mux1/2, y/1, Notch filter 1/1, Mux/1
  Mux/1 -> Scope/1
  Notch filter 3/1 -> Mux/4, q/1
  Notch filter 1/1 -> Mux/2, Notch filter 2/1
  Mux1/1 -> Scope1/1

== system Marine_LocoMotive_UAV_est_git/Sensors and Filters/Data processing/Estimate Position/2nd Order Filter ==
  u : Inport
  "  2" : Constant  Value=2
  "  wn" : Constant  Value=OMEGA_FILTER_OUTER
  "  zea" : Constant
  Discrete-Time Integrator : DiscreteIntegrator  SampleTime=-1  ICPrevOutput=DiscIntNeverNeededParam  ICPrevScaledInput=DiscIntNeverNeededParam
  Discrete-Time Integrator1 : DiscreteIntegrator  InitialCondition=X0_u(1)  SampleTime=-1  ICPrevOutput=DiscIntNeverNeededParam  ICPrevScaledInput=DiscIntNeverNeededParam
  Product : Product
  Product1 : Product
  Product2 : Product  Inputs=3
  Sum : Sum  Inputs=|+-
  Sum1 : Sum  Inputs=|+-
  y : Outport
  yd : Outport  Port=2
  wires:
  Sum/1 -> Sum1/1
  Discrete-Time Integrator/1 -> Product2/1, Product1/2
  Product/1 -> Discrete-Time Integrator/1
  "  wn"/1 -> Product1/1, Product/1
  Sum1/1 -> Product/2
  u/1 -> Sum/1
  Discrete-Time Integrator1/1 -> Sum/2, y/1
  Product1/1 -> Discrete-Time Integrator1/1, yd/1
  "  2"/1 -> Product2/2
  "  zea"/1 -> Product2/3
  Product2/1 -> Sum1/2

== system Marine_LocoMotive_UAV_est_git/Sensors and Filters/Data processing/Estimate Position/2nd Order Filter2 ==
  u : Inport
  "  2" : Constant  Value=2
  "  wn" : Constant  Value=OMEGA_FILTER_OUTER
  "  zea" : Constant
  Discrete-Time Integrator : DiscreteIntegrator  SampleTime=-1  ICPrevOutput=DiscIntNeverNeededParam  ICPrevScaledInput=DiscIntNeverNeededParam
  Discrete-Time Integrator1 : DiscreteIntegrator  InitialCondition=X0_u(2)  SampleTime=-1  ICPrevOutput=DiscIntNeverNeededParam  ICPrevScaledInput=DiscIntNeverNeededParam
  Product : Product
  Product1 : Product
  Product2 : Product  Inputs=3
  Sum : Sum  Inputs=|+-
  Sum1 : Sum  Inputs=|+-
  y : Outport
  yd : Outport  Port=2
  wires:
  Sum/1 -> Sum1/1
  Discrete-Time Integrator/1 -> Product2/1, Product1/2
  Product/1 -> Discrete-Time Integrator/1
  "  wn"/1 -> Product1/1, Product/1
  Sum1/1 -> Product/2
  u/1 -> Sum/1
  Discrete-Time Integrator1/1 -> Sum/2, y/1
  Product1/1 -> Discrete-Time Integrator1/1, yd/1
  "  2"/1 -> Product2/2
  "  zea"/1 -> Product2/3
  Product2/1 -> Sum1/2

== system Marine_LocoMotive_UAV_est_git/Sensors and Filters/Data processing/Estimate Position/2nd Order Filter4 ==
  u : Inport
  "  1" : Constant  Value=OMEGA_FILTER_OUTER
  "  2" : Constant  Value=2
  "  zea" : Constant
  Discrete-Time Integrator : DiscreteIntegrator  SampleTime=-1  ICPrevOutput=DiscIntNeverNeededParam  ICPrevScaledInput=DiscIntNeverNeededParam
  Discrete-Time Integrator1 : DiscreteIntegrator  InitialCondition=X0_u(2)  SampleTime=-1  ICPrevOutput=DiscIntNeverNeededParam  ICPrevScaledInput=DiscIntNeverNeededParam
  Product : Product
  Product1 : Product
  Product2 : Product  Inputs=3
  Sum : Sum  Inputs=|+-
  Sum1 : Sum  Inputs=|+-
  y : Outport
  yd : Outport  Port=2
  wires:
  Product2/1 -> Sum1/2
  "  zea"/1 -> Product2/3
  "  2"/1 -> Product2/2
  Product1/1 -> Discrete-Time Integrator1/1, yd/1
  Discrete-Time Integrator1/1 -> y/1, Sum/2
  u/1 -> Sum/1
  Sum1/1 -> Product/2
  "  1"/1 -> Product/1, Product1/1
  Product/1 -> Discrete-Time Integrator/1
  Discrete-Time Integrator/1 -> Product1/2, Product2/1
  Sum/1 -> Sum1/1

== system Marine_LocoMotive_UAV_est_git/Sensors and Filters/Data processing/Estimate Position/2nd Order Filter5 ==
  u : Inport
  "  2" : Constant  Value=2
  "  wn" : Constant  Value=OMEGA_FILTER_OUTER
  "  zea" : Constant
  Discrete-Time Integrator : DiscreteIntegrator  SampleTime=-1  ICPrevOutput=DiscIntNeverNeededParam  ICPrevScaledInput=DiscIntNeverNeededParam
  Discrete-Time Integrator1 : DiscreteIntegrator  InitialCondition=X0_u(2)  SampleTime=-1  ICPrevOutput=DiscIntNeverNeededParam  ICPrevScaledInput=DiscIntNeverNeededParam
  Product : Product
  Product1 : Product
  Product2 : Product  Inputs=3
  Sum : Sum  Inputs=|+-
  Sum1 : Sum  Inputs=|+-
  y : Outport
  yd : Outport  Port=2
  wires:
  Product2/1 -> Sum1/2
  "  zea"/1 -> Product2/3
  "  2"/1 -> Product2/2
  Product1/1 -> Discrete-Time Integrator1/1, yd/1
  Discrete-Time Integrator1/1 -> y/1, Sum/2
  u/1 -> Sum/1
  Sum1/1 -> Product/2
  "  wn"/1 -> Product/1, Product1/1
  Product/1 -> Discrete-Time Integrator/1
  Discrete-Time Integrator/1 -> Product1/2, Product2/1
  Sum/1 -> Sum1/1

== system Marine_LocoMotive_UAV_est_git/Sensors and Filters/Data processing/Estimate Position/Notch Filter2 ==
  u : Inport
  LPF : DiscreteTransferFcn  Numerator=Bm_LPF  Denominator=Am_LPF
  Mux : Mux  Commented=on  Inputs=3
  Notch filter : DiscreteTransferFcn  Numerator=an1_v  Denominator=bn1_v  SampleTime=Tn
  Scope : Scope  Commented=on
  y : Outport
  wires:
  Notch filter/1 -> y/1, Mux/3
  Mux/1 -> Scope/1
  LPF/1 -> Mux/2, Notch filter/1
  u/1 -> LPF/1, Mux/1

== system Marine_LocoMotive_UAV_est_git/Sensors and Filters/Data processing/Estimate Position/Signal Conditioning - Sonar ==
  note: Correct for Roll and Pitch
  sonar (m) : Inport
  pitch (rad) : Inport  Port=2
  "Height Estimate Bias (Estimate Reference at Centre of QBall 2) " : Bias
  Product : Product  RndMeth=Zero
  "The sonar signal is the true elevation, so no need for correction" : Constant
  Trigonometric Function : Trigonometry  Commented=on  Operator=cos
  calib sonar (m) : Outport
  wires:
  sonar (m)/1 -> Product/1
  pitch (rad)/1 -> Trigonometric Function/1
  "The sonar signal is the true elevation, so no need for correction"/1 -> Product/2
  Product/1 -> "Height Estimate Bias (Estimate Reference at Centre of QBall 2) "/1
  "Height Estimate Bias (Estimate Reference at Centre of QBall 2) "/1 -> calib sonar (m)/1

== system Marine_LocoMotive_UAV_est_git/Sensors and Filters/Sensors/ Sonar (10Hz) (true elevation instead real sonar signal)/FOH1 ==
  Input : Inport
  Bias : Bias  Bias=-Ts
  Constant : Constant
  Digital Clock : DigitalClock  DisableCoverage=on  SampleTime=Ts
  Discrete-Time Integrator : DiscreteIntegrator  SampleTime=-1  ICPrevOutput=DiscIntNeverNeededParam  ICPrevScaledInput=DiscIntNeverNeededParam
  Gain : Gain  DisableCoverage=on  Gain=1/Ts  SaturateOnIntegerOverflow=on  OutDataTypeStr=Inherit: Same as input  ParamDataTypeStr=Inherit: Same as input
  Product : Product  RndMeth=Zero
  Rate Transition : RateTransition
  Rate Transition1 : RateTransition  OutPortSampleTime=T
  Rate Transition3 : RateTransition  OutPortSampleTime=T
  Rate Transition4 : RateTransition  InitialCondition=X0_u(2)  OutPortSampleTime=Ts
  Rate Transition5 : RateTransition  OutPortSampleTime=T
  Scope : Scope  Commented=on
  Scope1 : Scope  Commented=on
  Sum : Sum  DisableCoverage=on  Inputs=|+-  SaturateOnIntegerOverflow=on  InputSameDT=on  OutDataTypeStr=Inherit: Same as first input
  Sum2 : Sum  DisableCoverage=on  Inputs=|+-  SaturateOnIntegerOverflow=on  InputSameDT=on  OutDataTypeStr=Inherit: Same as first input
  Unit Delay : UnitDelay  DisableCoverage=on  InitialCondition=X0_u(2)  SampleTime=Ts
  s : Sum  Inputs=++|  SaturateOnIntegerOverflow=on  InputSameDT=on  OutDataTypeStr=Inherit: Same as first input
  Output : Outport
  wires:
  Input/1 -> Rate Transition4/1, Rate Transition5/1
  Unit Delay/1 -> Sum/2
  Rate Transition1/1 -> Scope1/1, Product/1
  Product/1 -> s/2
  Rate Transition3/1 -> Product/2, Scope/1
  Sum/1 -> Rate Transition1/1
  Bias/1 -> Sum2/1
  Discrete-Time Integrator/1 -> Bias/1
  Rate Transition/1 -> Sum2/2
  s/1 -> Output/1
  Rate Transition5/1 -> s/1
  Gain/1 -> Rate Transition3/1
  Digital Clock/1 -> Rate Transition/1
  Sum2/1 -> Gain/1
  Constant/1 -> Discrete-Time Integrator/1
  Rate Transition4/1 -> Sum/1, Unit Delay/1

== system Marine_LocoMotive_UAV_est_git/Sensors and Filters/Sensors/ Sonar (10Hz) (true elevation instead real sonar signal)/Sampler ==
  In1 : Inport
  Constant : Constant  Value=X0_u(2)
  Derivative : Derivative
  Digital Clock : DigitalClock  DisableCoverage=on  SampleTime=0.1
  Rate Transition : RateTransition  InitialCondition=0.1
  Switch : Switch  Threshold=0.2
  Triggered Subsystem : Subsystem  TreatAsAtomicUnit=on
  Out1 : Outport
  wires:
  Derivative/1 -> Triggered Subsystem/Trigger
  Rate Transition/1 -> Derivative/1
  In1/1 -> Triggered Subsystem/1(In1)
  Switch/1 -> Out1/1
  Digital Clock/1 -> Switch/2, Rate Transition/1
  Triggered Subsystem/1(Out1) -> Switch/1
  Constant/1 -> Switch/3

== system Marine_LocoMotive_UAV_est_git/UAV controller/Coupling /Subsystem2/smooth switch ==
  u 1 : Inport
  u 2 : Inport  Port=2
  switch : Inport  Port=3
  Constant : Constant
  Data Type Conversion : DataTypeConversion
  Low Pass Filter2 : DiscreteTransferFcn  Numerator=Bm_coup_LPF  Denominator=Am_coup_LPF
  Product : Product
  Product1 : Product
  Subtract : Sum  Inputs=+-
  Sum : Sum  Inputs=|++
  "switch " : Scope
  y : Outport
  wires:
  Product/1 -> Sum/2
  Product1/1 -> Sum/1
  Low Pass Filter2/1 -> "switch "/1, Product/1, Subtract/2
  Data Type Conversion/1 -> Low Pass Filter2/1
  u 1/1 -> Product1/1
  u 2/1 -> Product/2
  switch/1 -> Data Type Conversion/1
  Sum/1 -> y/1
  Constant/1 -> Subtract/1
  Subtract/1 -> Product1/2

== system Marine_LocoMotive_UAV_est_git/UAV controller/Coupling /Subsystem3/smooth switch ==
  u 1 : Inport
  u 2 : Inport  Port=2
  switch : Inport  Port=3
  Constant : Constant
  Data Type Conversion : DataTypeConversion
  Low Pass Filter2 : DiscreteTransferFcn  Numerator=Bm_fast_coup_LPF  Denominator=Am_fast_coup_LPF
  Product : Product
  Product1 : Product
  Step1 : Step  SampleTime=0
  Subtract : Sum  Inputs=+-
  Sum : Sum  Inputs=|++
  "switch " : Scope
  y : Outport
  wires:
  Subtract/1 -> Product1/2
  Constant/1 -> Subtract/1
  Sum/1 -> y/1
  switch/1 -> Data Type Conversion/1
  u 2/1 -> Product/2
  u 1/1 -> Product1/1
  Data Type Conversion/1 -> Low Pass Filter2/1
  Low Pass Filter2/1 -> Subtract/2, Product/1, "switch "/1
  Product1/1 -> Sum/1
  Product/1 -> Sum/2

== system Marine_LocoMotive_UAV_est_git/UAV controller/Coupling /u_T switch/smooth switch ==
  u 1 : Inport
  u 2 : Inport  Port=2
  switch : Inport  Port=3
  Constant : Constant
  Data Type Conversion : DataTypeConversion
  Low Pass Filter2 : DiscreteTransferFcn  Numerator=Bm_fast_coup_LPF  Denominator=Am_fast_coup_LPF
  Product : Product
  Product1 : Product
  Step1 : Step  SampleTime=0
  Subtract : Sum  Inputs=+-
  Sum : Sum  Inputs=|++
  "switch " : Scope
  y : Outport
  wires:
  Product/1 -> Sum/2
  Product1/1 -> Sum/1
  Low Pass Filter2/1 -> "switch "/1, Product/1, Subtract/2
  Data Type Conversion/1 -> Low Pass Filter2/1
  u 1/1 -> Product1/1
  u 2/1 -> Product/2
  switch/1 -> Data Type Conversion/1
  Sum/1 -> y/1
  Constant/1 -> Subtract/1
  Subtract/1 -> Product1/2

== system Marine_LocoMotive_UAV_est_git/UAV controller/Coupling /u_a switch/smooth switch ==
  u 1 : Inport
  u 2 : Inport  Port=2
  switch : Inport  Port=3
  Constant : Constant
  Data Type Conversion : DataTypeConversion
  Low Pass Filter2 : DiscreteTransferFcn  Numerator=Bm_fast_coup_LPF  Denominator=Am_fast_coup_LPF
  Product : Product
  Product1 : Product
  Subtract : Sum  Inputs=+-
  Sum : Sum  Inputs=|++
  "switch " : Scope
  y : Outport
  wires:
  Subtract/1 -> Product1/2
  Constant/1 -> Subtract/1
  Sum/1 -> y/1
  switch/1 -> Data Type Conversion/1
  u 2/1 -> Product/2
  u 1/1 -> Product1/1
  Data Type Conversion/1 -> Low Pass Filter2/1
  Low Pass Filter2/1 -> Subtract/2, Product/1, "switch "/1
  Product1/1 -> Sum/1
  Product/1 -> Sum/2

== system Marine_LocoMotive_UAV_est_git/UAV controller/switch controllers/Smooth channel switching/C1 transition ==
  C1 : Inport
  switch : Inport  Port=2
  C2_0 : Inport  Port=3
  Compare To Constant : simulink/Logic and Bit Operations/Compare To Constant  relop=<  const=epsilon_e_u1  OutDataTypeStr=boolean
  Constant : Constant
  Constant1 : Constant  Value=epsilon_e_u1
  Delay1 : Delay  DelayLength=1
  IC : InitialCondition  Value=0
  Logical Operator : Logic  Operator=NOT  AllPortsSameDT=off  OutDataTypeStr=boolean
  Product : Product
  Subsystem : Subsystem
  Sum : Sum  Inputs=-+|
  Sum1 : Sum  Inputs=++|
  Sum3 : Sum  Inputs=|++
  Switch1 : Switch  Criteria=u2 > Threshold  Threshold=0.5
  Switch2 : Switch  Criteria=u2 > Threshold  Threshold=0.5
  latch : Subsystem  TreatAsAtomicUnit=on
  latch error ON : Scope
  record C2_0 : Subsystem  TreatAsAtomicUnit=on
  smooth transition to C1 : Subsystem  TreatAsAtomicUnit=on
  trigger and reset latch : Subsystem
  C1_trans : Outport
  wires:
  Sum1/1 -> Subsystem/1(addition with C2_0), Switch1/3  "addition with C2_0"
  C2_0/1 -> record C2_0/1(In1)
  smooth transition to C1/1(Out1) -> Sum1/2
  record C2_0/1(Out1) -> Sum/1, Sum1/1  "C2_0"
  C1/1 -> Subsystem/2(C1), Switch1/1, Sum/2  "C1"
  Switch1/1 -> C1_trans/1  "out"
  latch/1(Out1) -> Switch2/1
  Switch2/1 -> Switch1/2, latch error ON/1
  Constant/1 -> Switch2/3
  Constant1/1 -> Product/1
  Product/1 -> Sum3/2  "do not latch C1 is off"
  Sum3/1 -> Compare To Constant/1
  Subsystem/1(Out1) -> Sum3/1
  Compare To Constant/1 -> IC/1
  Delay1/1 -> smooth transition to C1/2(reset)
  Sum/1 -> smooth transition to C1/1(In1)
  switch/1 -> Switch2/2, Logical Operator/1, Delay1/1, record C2_0/Trigger, trigger and reset latch/1(In1), Subsystem/Enable, smooth transition to C1/Enable
  IC/1 -> trigger and reset latch/2(In2), latch/1(In1)
  Logical Operator/1 -> Product/2
  trigger and reset latch/1(Out1) -> latch/Trigger

== system Marine_LocoMotive_UAV_est_git/UAV controller/switch controllers/Smooth channel switching/C2 transition ==
  C2 : Inport
  switch : Inport  Port=2
  C1_0 : Inport  Port=3
  Compare To Constant : simulink/Logic and Bit Operations/Compare To Constant  relop=<  const=epsilon_e_u1  OutDataTypeStr=boolean
  Constant : Constant
  Constant1 : Constant  Value=epsilon_e_u1
  Delay1 : Delay  DelayLength=1
  Logical Operator : Logic  Operator=NOT  AllPortsSameDT=off  OutDataTypeStr=boolean
  Product : Product
  Subsystem : Subsystem
  Sum : Sum  Inputs=-+|
  Sum1 : Sum  Inputs=++|
  Sum3 : Sum  Inputs=|++
  Switch1 : Switch  Criteria=u2 > Threshold  Threshold=0.5
  Switch2 : Switch  Criteria=u2 > Threshold  Threshold=0.5
  latch : Subsystem  TreatAsAtomicUnit=on
  latch error ON : Scope
  record C1_0 : Subsystem  TreatAsAtomicUnit=on
  smooth transition to C1 : Subsystem  TreatAsAtomicUnit=on
  trigger and reset latch : Subsystem
  C2_trans : Outport
  wires:
  Sum/1 -> smooth transition to C1/1(In1)
  Switch1/1 -> C2_trans/1  "out"
  C2/1 -> Sum/2, Subsystem/2(C2), Switch1/1  "C2"
  Switch2/1 -> Switch1/2, latch error ON/1
  switch/1 -> Switch2/2, Logical Operator/1, Delay1/1, smooth transition to C1/Enable, Subsystem/Enable, trigger and reset latch/1(trigger), record C1_0/Trigger  "trigger"
  record C1_0/1(Out1) -> Sum1/1, Sum/1  "C1_0"
  smooth transition to C1/1(Out1) -> Sum1/2
  C1_0/1 -> record C1_0/1(In1)
  Sum1/1 -> Subsystem/1(addition with C1_0), Switch1/3  "addition with C1_0"
  Constant/1 -> Switch2/3
  latch/1(Out1) -> Switch2/1
  Product/1 -> Sum3/2
  Constant1/1 -> Product/1
  Sum3/1 -> Compare To Constant/1
  Logical Operator/1 -> Product/2
  Delay1/1 -> smooth transition to C1/2(reset)
  Subsystem/1(Out1) -> Sum3/1
  Compare To Constant/1 -> trigger and reset latch/2(In2), latch/1(In1)
  trigger and reset latch/1(Out1) -> latch/Trigger

== system Marine_LocoMotive_UAV_est_git/UAV controller/u_a_Lyapunov/Subsystem1/Enabled Subsystem1 ==
  u : Inport
  reset : Inport  Port=2
  u0 : Inport  Port=3
  Enable : EnablePort
  Logical Operator : Logic  Operator=NOT  AllPortsSameDT=off  OutDataTypeStr=boolean
  Low Pass Filter5 : DiscreteTransferFcn  Numerator=Bm_rdeL_LPF  Denominator=Am_rdeL_LPF  InitialStatesSource=Input port  ExternalReset=Level
      settings: InputPortMap=u0,r7,p5
  Mux2 : Mux  Inputs=2
  adjustment for this specific transfer function : Gain  Gain=84.6505602
  r_dot filt : Scope
  r_dot filt1 : Scope
  y : Outport
  wires:
  u/1 -> Mux2/2, Low Pass Filter5/1
  Low Pass Filter5/1 -> Mux2/1, y/1
  Logical Operator/1 -> r_dot filt1/1, Low Pass Filter5/2
  u0/1 -> adjustment for this specific transfer function/1
  Mux2/1 -> r_dot filt/1
  adjustment for this specific transfer function/1 -> Low Pass Filter5/3
  reset/1 -> Logical Operator/1
